simulink model "Last_EKFForAVehicle_SimulinkModel"  (R2019b)
settings: Solver=FixedStepDiscrete  StartTime=0.0  StopTime=TFinal  FixedStep=Ts  RelTol=1e-3
values from neighbouring files (symbols this model uses):
  cx = 2    [Test_EKF_circular_trajectory.m]
  cy = 2    [Test_EKF_circular_trajectory.m]
  muWx = 0    [Test_EKF_circular_trajectory.m]
  muWy = 0    [Test_EKF_circular_trajectory.m]
  P0 = [1;1]    [Test_EKF_circular_trajectory.m]
  sigB = 1e-1    (= 0.1)    [Test_EKF_circular_trajectory.m]
  sigR = 1e-1    (= 0.1)    [Test_EKF_circular_trajectory.m]
  sigWx = 1e-7    (= 1e-07)    [Test_EKF_circular_trajectory.m]
  sigWy = 1e-7    (= 1e-07)    [Test_EKF_circular_trajectory.m]
  Ts = 0.01    [KF_Pendulum_parameter.m]    (also in Test_EKF_circular_trajectory.m)
  V0 = [-0.25;0.25]    [Test_EKF_circular_trajectory.m]
  wx = 0    [Test_EKF_circular_trajectory.m]
  wy = 0    [Test_EKF_circular_trajectory.m]
  Z = 2    [Test_EKF_circular_trajectory.m]
undefined symbols (not defined in the file or in its folder): randraw
settings Model: Creator=starl  LastModifiedBy=starl

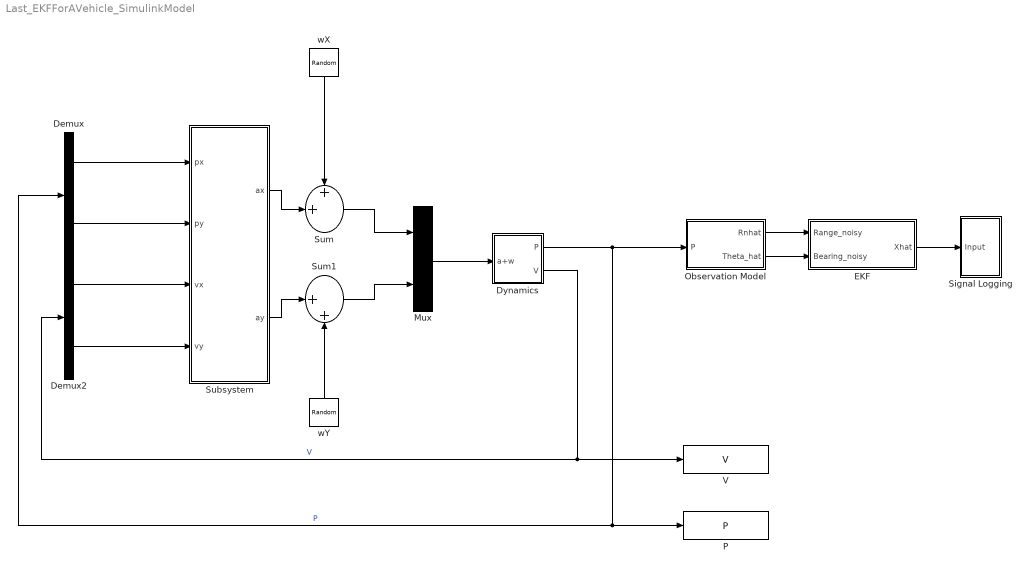
== system Last_EKFForAVehicle_SimulinkModel ==
  Demux : Demux  Outputs=2
  Demux2 : Demux  Outputs=2
  Dynamics : Subsystem
  EKF : Subsystem
  Mux : Mux  Inputs=2
  Observation Model : Subsystem
  P : ToWorkspace  VariableName=P  SampleTime=-1
  Signal Logging : Subsystem
  Subsystem : Subsystem
  Sum : Sum  Inputs=++|
  Sum1 : Sum  Inputs=|++
  V : ToWorkspace  VariableName=V  SampleTime=-1
  wX : RandomNumber  Mean=muWx  Variance=sigWx  Seed=2^wx  SampleTime=Ts
  wY : RandomNumber  Mean=muWy  Variance=sigWy  Seed=2^wy  SampleTime=Ts
  wires:
  Demux/2 -> Subsystem/2("py ")
  Demux/1 -> Subsystem/1(px)
  Demux2/1 -> Subsystem/3(vx)
  Demux2/2 -> Subsystem/4(vy)
  Subsystem/1(ax) -> Sum/2
  wY/1 -> Sum1/2
  wX/1 -> Sum/1
  Subsystem/2(ay) -> Sum1/1
  Mux/1 -> Dynamics/1(a+w)
  Dynamics/1(P) -> Observation Model/1(P), P/1, Demux/1  "P"
  Dynamics/2(V) -> V/1, Demux2/1  "V"
  Observation Model/2(Theta_hat) -> EKF/2(Bearing_noisy)
  Observation Model/1(Rnhat) -> EKF/1(Range_noisy)
  EKF/1(Xhat) -> Signal Logging/1(Input)
  Sum/1 -> Mux/1
  Sum1/1 -> Mux/2

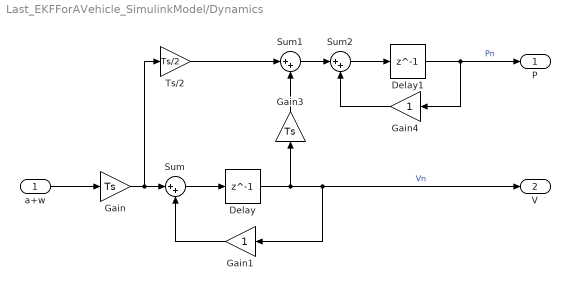
== system Last_EKFForAVehicle_SimulinkModel/Dynamics ==
  a+w : Inport
  Delay : Delay  DelayLength=1  InitialCondition=0
  Delay1 : Delay  DelayLength=1  InitialCondition=0
  Gain : Gain  Gain=Ts
  Gain1 : Gain
  Gain3 : Gain  Gain=Ts
  Gain4 : Gain
  Sum : Sum  Inputs=|++
  Sum1 : Sum  Inputs=|++
  Sum2 : Sum  Inputs=|++
  Ts/2 : Gain  Gain=Ts/2
  P : Outport
  V : Outport  Port=2
  wires:
  Sum/1 -> Delay/1
  Delay/1 -> V/1, Gain1/1, Gain3/1  "Vn"
  Gain1/1 -> Sum/2
  Delay1/1 -> P/1, Gain4/1  "Pn"
  Gain/1 -> Ts/2/1, Sum/1
  a+w/1 -> Gain/1
  Gain3/1 -> Sum1/2
  Gain4/1 -> Sum2/2
  Ts/2/1 -> Sum1/1
  Sum2/1 -> Delay1/1
  Sum1/1 -> Sum2/1

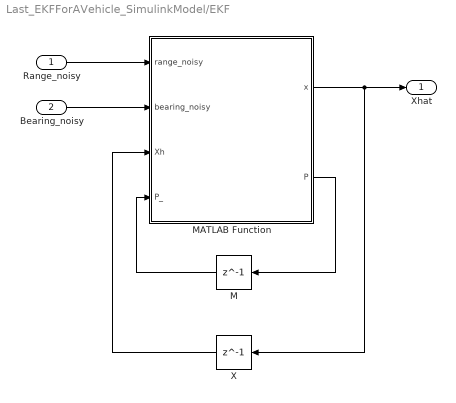
== system Last_EKFForAVehicle_SimulinkModel/EKF ==
  Range_noisy : Inport
  Bearing_noisy : Inport  Port=2
  M : Delay  DelayLength=1  InitialCondition=zeros(4,4)
  MATLAB Function : MATLAB Function  TreatAsAtomicUnit=on
  X : Delay  DelayLength=1  InitialCondition=[P0;V0]
  Xhat : Outport
  wires:
  MATLAB Function/1(x) -> Xhat/1, X/1
  M/1 -> MATLAB Function/4(P_)
  Bearing_noisy/1 -> MATLAB Function/2(bearing_noisy)
  MATLAB Function/2(P) -> M/1
  X/1 -> MATLAB Function/3(Xh)
  Range_noisy/1 -> MATLAB Function/1(range_noisy)

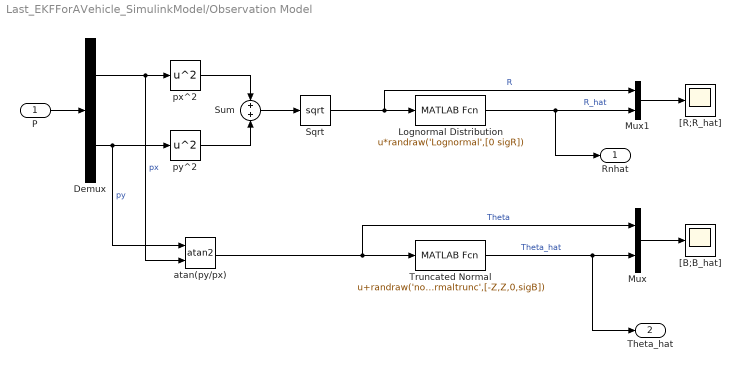
== system Last_EKFForAVehicle_SimulinkModel/Observation Model ==
  P : Inport
  Demux : Demux  Outputs=2
  "Lognormal Distribution " : MATLABFcn  MATLABFcn=u*randraw('Lognormal',[0 sigR])
  Mux : Mux  Inputs=2
  Mux1 : Mux  Inputs=2
  Sqrt : Sqrt  SaturateOnIntegerOverflow=on
  Sum : Sum  Inputs=+|+
  Truncated Normal : MATLABFcn  MATLABFcn=u+randraw('normaltrunc',[-Z,Z,0,sigB])
  "[B;B_hat]" : Scope
  "[R;R_hat]" : Scope
  atan(py/px) : Trigonometry  Operator=atan2
  px^2 : Math  Operator=square  SignedPower=off  SaturateOnIntegerOverflow=on
  py^2 : Math  Operator=square  SignedPower=off  SaturateOnIntegerOverflow=on
  Rnhat : Outport
  Theta_hat : Outport  Port=2
  wires:
  Demux/1 -> atan(py/px)/2, px^2/1  "px"
  py^2/1 -> Sum/2
  Sqrt/1 -> Mux1/1, "Lognormal Distribution "/1  "R"
  atan(py/px)/1 -> Mux/1, Truncated Normal/1  "Theta"
  P/1 -> Demux/1
  Sum/1 -> Sqrt/1
  Truncated Normal/1 -> Theta_hat/1, Mux/2  "Theta_hat"
  "Lognormal Distribution "/1 -> Rnhat/1, Mux1/2  "R_hat"
  Mux/1 -> "[B;B_hat]"/1
  px^2/1 -> Sum/1
  Mux1/1 -> "[R;R_hat]"/1
  Demux/2 -> atan(py/px)/1, py^2/1  "py"

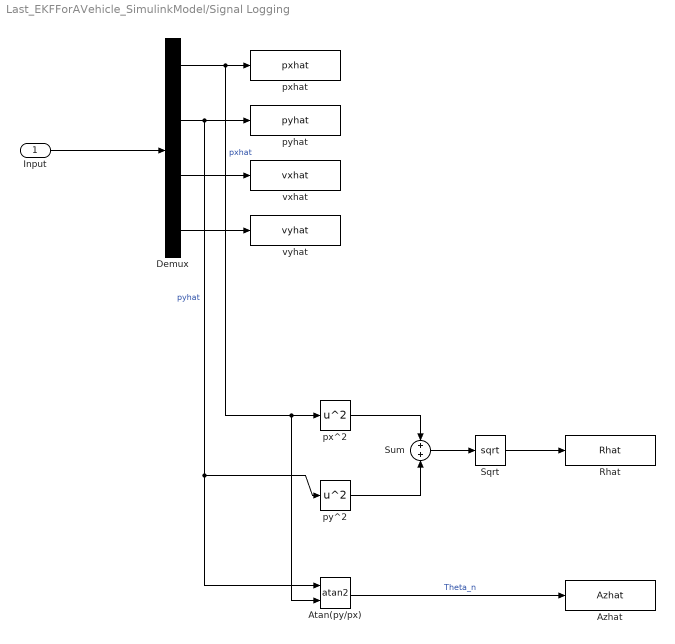
== system Last_EKFForAVehicle_SimulinkModel/Signal Logging ==
  Input : Inport
  Atan(py/px) : Trigonometry  Operator=atan2
  Azhat : ToWorkspace  VariableName=Azhat  SampleTime=-1
  Demux : Demux
  Rhat : ToWorkspace  VariableName=Rhat  SampleTime=-1
  Sqrt : Sqrt  SaturateOnIntegerOverflow=on
  Sum : Sum  Inputs=+|+
  px^2 : Math  Operator=square  SignedPower=off  SaturateOnIntegerOverflow=on
  pxhat : ToWorkspace  VariableName=pxhat  SampleTime=-1
  py^2 : Math  Operator=square  SignedPower=off  SaturateOnIntegerOverflow=on
  pyhat : ToWorkspace  VariableName=pyhat  SampleTime=-1
  vxhat : ToWorkspace  VariableName=vxhat  SampleTime=-1
  vyhat : ToWorkspace  VariableName=vyhat  SampleTime=-1
  wires:
  Demux/2 -> Atan(py/px)/1, py^2/1, pyhat/1  "pyhat"
  Demux/1 -> Atan(py/px)/2, px^2/1, pxhat/1  "pxhat"
  px^2/1 -> Sum/1
  Sqrt/1 -> Rhat/1
  py^2/1 -> Sum/2
  Demux/3 -> vxhat/1
  Input/1 -> Demux/1
  Atan(py/px)/1 -> Azhat/1  "Theta_n"
  Demux/4 -> vyhat/1
  Sum/1 -> Sqrt/1

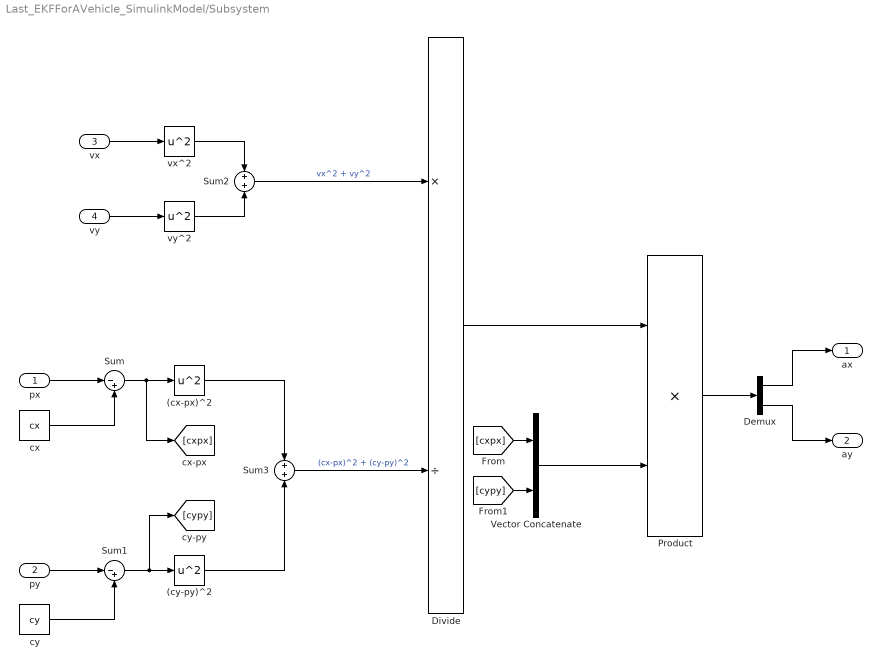
== system Last_EKFForAVehicle_SimulinkModel/Subsystem ==
  px : Inport
  "py " : Inport  Port=2
  vx : Inport  Port=3
  vy : Inport  Port=4
  (cx-px)^2 : Math  Operator=square  SignedPower=off  SaturateOnIntegerOverflow=on
  (cy-py)^2 : Math  Operator=square  SignedPower=off  SaturateOnIntegerOverflow=on
  Demux : Demux  Outputs=2
  Divide : Product  Inputs=*/
  Product : Product
  Sum : Sum  Inputs=|-+
  Sum1 : Sum  Inputs=|-+
  Sum2 : Sum  Inputs=+|+
  Sum3 : Sum  Inputs=+|+
  Vector Concatenate : Concatenate
  "cx " : Constant  Value=cx
  cy : Constant  Value=cy
  vx^2 : Math  Operator=square  SignedPower=off  SaturateOnIntegerOverflow=on
  vy^2 : Math  Operator=square  SignedPower=off  SaturateOnIntegerOverflow=on
  ax : Outport
  ay : Outport  Port=2
  wires:
  vy^2/1 -> Sum2/2
  vx^2/1 -> Sum2/1
  [cxpx] -> Vector Concatenate/1
  vy/1 -> vy^2/1
  Sum3/1 -> Divide/2  "(cx-px)^2 + (cy-py)^2"
  Sum2/1 -> Divide/1  "vx^2 + vy^2"
  Sum/1 -> [cxpx], (cx-px)^2/1
  "cx "/1 -> Sum/2
  "py "/1 -> Sum1/1
  Demux/2 -> ay/1
  Product/1 -> Demux/1
  Vector Concatenate/1 -> Product/2
  Sum1/1 -> [cypy], (cy-py)^2/1
  px/1 -> Sum/1
  [cypy] -> Vector Concatenate/2
  cy/1 -> Sum1/2
  Demux/1 -> ax/1
  (cx-px)^2/1 -> Sum3/1
  vx/1 -> vx^2/1
  (cy-py)^2/1 -> Sum3/2
  Divide/1 -> Product/1

== matlab function Last_EKFForAVehicle_SimulinkModel/EKF/MATLAB Function ==
  data: range_noisy input; x output; bearing_noisy input; Xh input; P_ input; P output
function [x,P] = EKF(range_noisy,bearing_noisy,Xh,P_)

Ts = 1/100;

sigWx = 1e-7;
sigWy = 1e-7;

sigR = 1e-1;
sigB = 1e-1;
Q = [sigWx 0;0 sigWy];
R = [sigB 0;0 sigB];

cx = 2;
cy = 2;

px = Xh(1);
py = Xh(2);
vx = Xh(3);
vy = Xh(4);

A= Ajacob(cx,cy,px,py,vx,vy,Ts);
L = Lmat(Ts);

Pos = [px;py];
Vel = [vx;vy];

ax = ((vx^2 + vy^2)*(cx - px))/((cx-px)^2 + (cy-py)^2);
ay = ((vx^2 + vy^2)*(cy - py))/((cx-px)^2 + (cy-py)^2);

alph = [ax;ay];

xp = [Pos;zeros(2,1)] + [Ts*Vel;Vel] + Ts*[zeros(2,1);alph] + ((Ts^2)/2)*[alph;zeros(2,1)];
Pp = A*P_*A' + L*Q*L';

pxup = xp(1);
pyup = xp(2);
vxup = xp(3);
vyup = xp(4);

H = Hjacob(pxup,pyup);
M = Mjacob(pxup,pyup);

K = Pp*H'*inv(H*Pp*H' + M*R*M');
x = xp + K*([range_noisy;bearing_noisy] - [(xp(1)^2 + xp(2)^2) ^0.5;atan2(xp(2),xp(1))]);
P = (eye(4) - K*H)*Pp;
end

function A = Ajacob(cx,cy,px,py,vx,vy,Ts)
a = (cx-px)^2 + (cy-py)^2;
b = vx^2 + vy^2;
c= b/a;

a11 = 1+c*((cx-px)^2/a - (1/2))*Ts^2;
a12 = c*(1/a)*(cx-px)*(cy-py)*Ts^2;
a13 = (1/a)*vx*(cx-px)*Ts^2;
a14 = (1/a)*vy*(cy-py)*Ts^2;

a21 = c*(1/a)*(cx-px)*(cy-py)*Ts^2;
a22 = 1+(Ts^2*c*((1/a)*(cy-py)^2 - (1/2)));
a23 = (Ts/a)*(vx*(cy-py));
a24 =Ts + ((vy/a)*(cy-py))*Ts^2;

a31 = c*(Ts*(2/a)*(cx-px)^2-Ts);
a32 = (2*Ts*c)*(1/a)*(cy-py)*(cx-px);
a33 = 1+(2*Ts/a)*vx*(cx-px);
a34 = (2*Ts/a)*vy*(cx-px);

a41 = 2*(c/a)*(cx-px)*(cy-py);
a42 = c*((2/a)*(cy-py)^2 - 1)*Ts;
a43 = (2*Ts/a)*vx*(cy-py);
a44 = 1+(2*Ts/a)*(cy-py);

A = [a11 a12 a13 a14;
     a21 a22 a23 a24;
     a31 a32 a33 a34;
     a41 a42 a43 a44];
end

function L = Lmat(Ts)

l11 = (Ts^2)/2;
l12 =0;
l21 =0;
l22 =l11;
l31 =Ts;
l32 =0;
l41 =0;
l42 =Ts;

L = [l11 l12; l21 l22; l31 l32; l41 l42];
end

function H = Hjacob(pxup,pyup)

H = [0 0 0 0; -pyup/(pxup^2 + pyup^2) , pxup/(pxup^2 + pyup^2), 0, 0];
end

function M = Mjacob(pxup,pyup)

M = [(pxup^2 + pyup^2)^(1/2),0 ; 0,1];
end
